simulink model "rozdzielacz_implementacja"  (R2022a)
settings: Solver=ode3  StartTime=0  StopTime=T_symulacji  FixedStep=T_probkowania  RelTol=1e-3
values from neighbouring files (symbols this model uses):
  k = 0.9    [Realizacja_sterowania.m]
  T_probkowania = 0.1    [Realizacja_sterowania.m]
  tryb = 1    [Realizacja_sterowania.m]
  V0 = 150    [Realizacja_sterowania.m]
undefined symbols (not defined in the file or in its folder): National_Instruments, PCIe, rozdzielacz
libraries: sldrtlib x5
settings Model: Creator=Jarek  LastModifiedBy=student
settings SolverCC: AlgebraicLoopSolver=TrustRegion
settings DataIOCC: LimitDataPoints=on  SaveFormat=Array  SignalLoggingSaveFormat=ModelDataLogs  ReturnWorkspaceOutputs=off
settings OptimizationCC: ExpressionDepthLimit=2147483647
settings DebuggingCC: UnderspecifiedInitializationDetection=Classic  MergeDetectMultiDrivingBlocksExec=none  SolverPrmCheckMsg=warning  FcnCallInpInsideContextMsg=warning  UnconnectedInputMsg=warning  UnconnectedOutputMsg=warning  UnconnectedLineMsg=warning  StateNameClashWarn=warning  SFUnexpectedBacktrackingDiag=warning  SFNoUnconditionalDefaultTransitionDiag=warning  SFExecutionAtInitializationDiag=none  ArithmeticOperatorsInVariantConditions=warning
settings HardwareCC: ProdBitPerLong=64  ProdHWDeviceType=Intel->x86-64 (Linux 64)
settings ModelReferenceCC: EnableRefExpFcnMdlSchedulingChecks=off  PropagateSignalLabelsOutOfModel=off
settings SFSimCC: SimUseLocalCustomCode=off  CustomCodeUndefinedFunction=UseInterfaceOnly
settings RTWCC: Description=Simulink Desktop Real-Time  SystemTargetFile=sldrt.tlc  TemplateMakefile=sldrt.tmf  RTWUseLocalCustomCode=off  RTWCompilerOptimization=on
settings CodeAppCC: MaxIdLength=95  StateflowObjectComments=on
settings SimulinkDesktopRealTimeCC: TargetLibSuffix=_sldrt.a  TargetPreCompLibLocation=C:\Program Files\MATLAB\R2022a\toolbox\sldrt\lib\win64  ParMdlRefBuildCompliant=on
settings ConfigComp: CovMetricSettings=dw  CovSaveCumulativeToWorkspaceVar=on  CovSaveSingleToWorkspaceVar=on  CovExternalEMLEnable=off

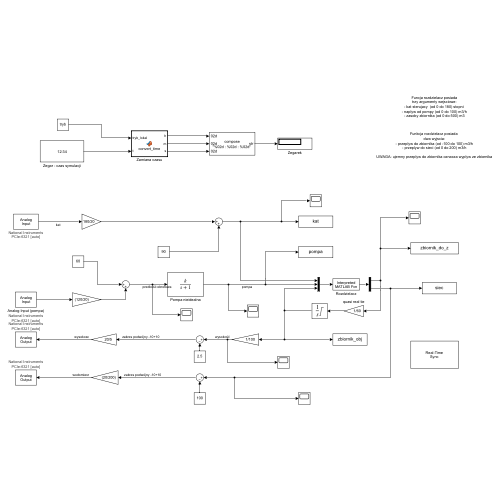
[thumbnail: Simulink's stored preview of the top-level diagram]
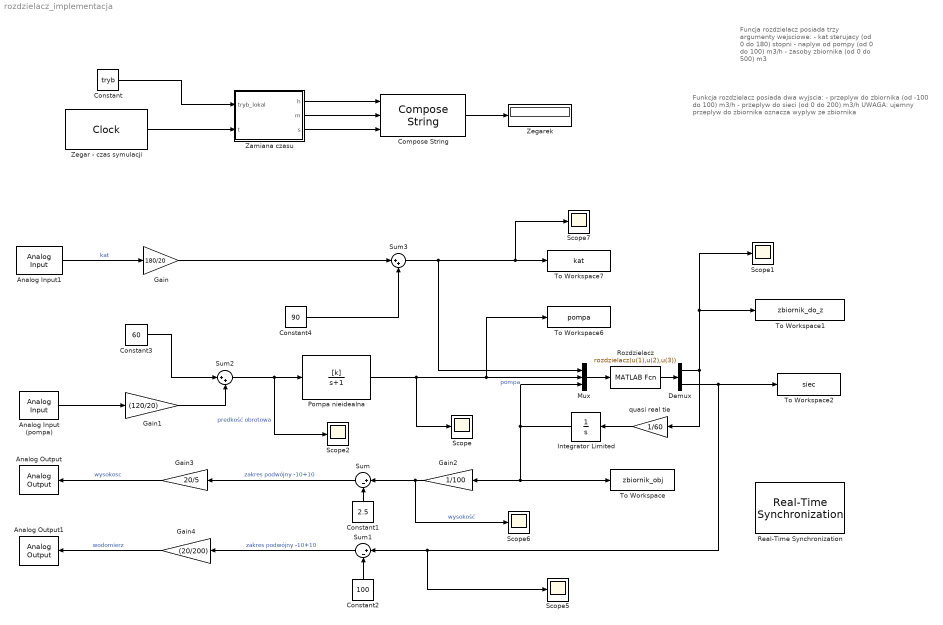
== system rozdzielacz_implementacja ==
  note: Funcja rozdzielacz posiada
      | trzy argumenty wejsciowe:
      | - kat sterujacy  (od 0 do 180) stopni
      | - naplyw od pompy (od 0 do 100) m3/h
      | - zasoby zbiornika (od 0 do 500) m3
  note: Funkcja rozdzielacz posiada
      | dwa wyjscia:
      | - przeplyw do zbiornika (od -100 do 100) m3/h
      | - przeplyw do sieci (od 0 do 200) m3/h
      |
      | UWAGA: ujemny przeplyw do zbiornika oznacza wyplyw ze zbiornika
  Analog Input (pompa) : sldrtlib/Analog Input  SampleTime=0.1  MaxMissedTicks=10  ShowMissedTicks=off  YieldWhenWaiting=off  DrvName=National_Instruments/PCIe-6321  DrvAddress=4294967295  DrvOptions=[0 0 0 0 0 0 0]  Channels=1  RangeMode=1  VoltRange=1  DataType=1
      settings: AttributesFormatString=National Instruments\nPCIe-6321 [auto]
  Analog Input1 : sldrtlib/Analog Input  SampleTime=0.1  MaxMissedTicks=10  ShowMissedTicks=off  YieldWhenWaiting=off  DrvName=National_Instruments/PCIe-6321  DrvAddress=4294967295  DrvOptions=[0 0 0 0 0 0 0]  Channels=2  RangeMode=1  VoltRange=1  DataType=1
      settings: AttributesFormatString=National Instruments\nPCIe-6321 [auto]
  Analog Output : sldrtlib/Analog Output  SampleTime=0.1  MaxMissedTicks=10  ShowMissedTicks=off  YieldWhenWaiting=off  DrvName=National_Instruments/PCIe-6321  DrvAddress=4294967295  DrvOptions=[0 0 0 0 0 0 0]  Channels=1  RangeMode=1  VoltRange=1  InitialValue=[]  FinalValue=[]
      settings: AttributesFormatString=National Instruments\nPCIe-6321 [auto]
  Analog Output1 : sldrtlib/Analog Output  SampleTime=0.1  MaxMissedTicks=10  ShowMissedTicks=off  YieldWhenWaiting=off  DrvName=National_Instruments/PCIe-6321  DrvAddress=4294967295  DrvOptions=[0 0 0 0 0 0 0]  Channels=2  RangeMode=1  VoltRange=1  InitialValue=[]  FinalValue=[]
      settings: AttributesFormatString=National Instruments\nPCIe-6321 [auto]
  Compose String : ComposeString  Format="\"%02d : %02d : %02d\""
  Constant : Constant  Value=tryb
  Constant1 : Constant  Value=2.5
  Constant2 : Constant  Value=100
  Constant3 : Constant  Value=60
  Constant4 : Constant  Value=90
  Demux : Demux  Outputs=2
  Gain : Gain  Gain=180/20
  Gain1 : Gain  Gain=(120/20)
  Gain2 : Gain  Gain=1/100
  Gain3 : Gain  Gain=20/5
  Gain4 : Gain  Gain=(20/200)
  Integrator Limited : Integrator  InitialCondition=V0  LimitOutput=on  UpperSaturationLimit=500  LowerSaturationLimit=0
  Mux : Mux  Inputs=3
  Pompa nieidealna : TransferFcn  Numerator=[k]  Denominator=[1 1]
  Real-Time Synchronization : sldrtlib/Real-Time Synchronization  SampleTime=T_probkowania  MaxMissedTicks=20  ShowMissedTicks=off  YieldWhenWaiting=off
  Rozdzielacz : MATLABFcn  MATLABFcn=rozdzielacz(u(1),u(2),u(3))  OutputDimensions=2
  Scope{,1..2,5..7} (6 alike) : Scope
  Sum : Sum  Inputs=|+-
  Sum1 : Sum  Inputs=|+-
  Sum2 : Sum  Inputs=|++
  Sum3 : Sum  Inputs=|++
  To Workspace : ToWorkspace  VariableName=zbiornik_obj  SaveFormat=Timeseries  SampleTime=T_probkowania
  To Workspace1 : ToWorkspace  VariableName=zbiornik_do_z  SaveFormat=Timeseries  SampleTime=T_probkowania
  To Workspace2 : ToWorkspace  VariableName=siec  SaveFormat=Timeseries  SampleTime=T_probkowania
  To Workspace6 : ToWorkspace  VariableName=pompa  SaveFormat=Timeseries  SampleTime=T_probkowania
  To Workspace7 : ToWorkspace  VariableName=kat  SaveFormat=Timeseries  SampleTime=T_probkowania
  Zamiana czasu : MATLAB Function  TreatAsAtomicUnit=on
  Zegar - czas symulacji : DigitalClock  SampleTime=T_probkowania
  Zegarek : Display
  quasi real tie : Gain  Gain=1/60
  wires:
  Mux/1 -> Rozdzielacz/1
  Rozdzielacz/1 -> Demux/1
  Demux/1 -> Scope1/1, To Workspace1/1, quasi real tie/1
  Integrator Limited/1 -> Mux/3, To Workspace/1, Gain2/1
  Demux/2 -> Scope5/1, Sum1/1, To Workspace2/1
  Sum3/1 -> Mux/1, Scope7/1, To Workspace7/1
  Zegar - czas symulacji/1 -> Zamiana czasu/2(t)
  Zamiana czasu/1(h) -> Compose String/1
  Zamiana czasu/2(m) -> Compose String/2
  Zamiana czasu/3(s) -> Compose String/3
  Compose String/1 -> Zegarek/1
  Constant/1 -> Zamiana czasu/1(tryb_lokal)
  Sum/1 -> Gain3/1  "zakres podwójny -10+10"
  Gain2/1 -> Scope6/1, Sum/1  "wysokość"
  Constant1/1 -> Sum/2
  Constant2/1 -> Sum1/2
  Sum1/1 -> Gain4/1  "zakres podwójny -10+10"
  Analog Input (pompa)/1 -> Gain1/1
  Gain1/1 -> Sum2/2
  Constant3/1 -> Sum2/1
  Analog Input1/1 -> Gain/1  "kat"
  Gain/1 -> Sum3/1
  Constant4/1 -> Sum3/2
  quasi real tie/1 -> Integrator Limited/1
  Sum2/1 -> Scope2/1, Pompa nieidealna/1  "predkość obrotowa"
  Pompa nieidealna/1 -> Scope/1, To Workspace6/1, Mux/2  "pompa"
  Gain4/1 -> Analog Output1/1  "wodomierz"
  Gain3/1 -> Analog Output/1  "wysokosc"

== matlab function rozdzielacz_implementacja/Zamiana czasu ==
  data: tryb_lokal input; t input; h output; m output; s output
function [h, m, s] = convert_time(tryb_lokal, t)
    switch tryb_lokal
    case 1
        t = t * 60;
    case 2
        t = t * 600;
    case 3
        t = t * 3600;
    end

    h = int32(floor(t / 3600));
    m = int8(floor(mod(t, 3600) / 60));
    s = int8(floor(mod(t, 60)));
end
